simulink model "BikeManualControl"  (R2023b)
settings: Solver=VariableStepAuto  StartTime=0.0  StopTime=20  RelTol=1e-3
InitFcn:
  | run("config.m")
  | run("tracks\track_loader.mlx")
values from neighbouring files (symbols this model uses):
  angleFF = (lambda)    [INIT_BlueBike.m]    (also in config.m)
  angleRF = angleRF * (180/pi)    [INIT_BlueBike.m]    (also in config.m)
  b_contact_RW = 2e3    (= 2000)    [INIT_BlueBike.m]    (also in config.m)
  C_F_alpha = 1e3    (= 1000)    [INIT_BlueBike.m]    (also in config.m)
  C_F_kappa = 1e3    (= 1000)    [INIT_BlueBike.m]    (also in config.m)
  CM_phi = 0.3    [INIT_BlueBike.m]    (also in config.m)
  Dtheta0 = v0 / radiusRW    (= 0)    [INIT_BlueBike.m]    (also in config.m)
  Dtheta0_FW = v0 / radiusFW    (= 0)    [INIT_BlueBike.m]    (also in config.m)
  epsilon = 1e-2    (= 0.01)    [INIT_BlueBike.m]    (also in config.m)
  g = 9.81    [INIT_BlueBike.m]    (also in config.m)
  isoCameraAimX = (1/2)*w + 0.75    (= 1.267)    [INIT_BlueBike.m]    (also in config.m)
  isoCameraX = -2    [INIT_BlueBike.m]    (also in config.m)
  isoCameraY = -1.0    (= -1)    [INIT_BlueBike.m]    (also in config.m)
  isoCameraZ = -2*w    (= -2.068)    [INIT_BlueBike.m]    (also in config.m)
  k_contact_FW = 1e5    (= 100000)    [INIT_BlueBike.m]    (also in config.m)
  k_contact_RW = 1e5    (= 100000)    [INIT_BlueBike.m]    (also in config.m)
  lengthFF = frontHinge / (sind(lambda))    [INIT_BlueBike.m]    (also in config.m)
  lengthRF = sqrt((w-frontHinge)^2 + adj^2)    [INIT_BlueBike.m]    (also in config.m)
  lengthRW = 0.03    [INIT_BlueBike.m]    (also in config.m)
  massRW = 2    [INIT_BlueBike.m]    (also in config.m)
  max_rw_t = 10.0    (= 10)    [INIT_BlueBike.m]    (also in config.m = 20)
  max_steer_t = 5.0    (= 5)    [INIT_BlueBike.m]    (also in config.m)
  mB = 15    [INIT_BlueBike.m]    (also in config.m)
  mH = 5    [INIT_BlueBike.m]    (also in config.m)
  radiusFW = 0.325    [INIT_BlueBike.m]    (also in config.m)
  radiusRW = 0.32    [INIT_BlueBike.m]    (also in config.m)
  sigma = 0.12    [INIT_BlueBike.m]    (also in config.m)
  topViewX = -4.5*w    (= -4.653)    [INIT_BlueBike.m]    (also in config.m)
  topViewY = 0*w    (= 0)    [INIT_BlueBike.m]    (also in config.m)
  topViewZ = 1*w    (= 1.034)    [INIT_BlueBike.m]    (also in config.m)
  xPla = 3e3    (= 3000)    [INIT_BlueBike.m]    (also in config.m)
  yPla = 3e3    (= 3000)    [INIT_BlueBike.m]    (also in config.m)
  zPla = 0.01    [INIT_BlueBike.m]    (also in config.m)
undefined symbols (not defined in the file or in its folder): Cylinder, Parts_Lib, X, Y, Z
libraries: sm_lib x78, nesl_utility x32, vrlib x14, simulink x3
(part 4 of 4)

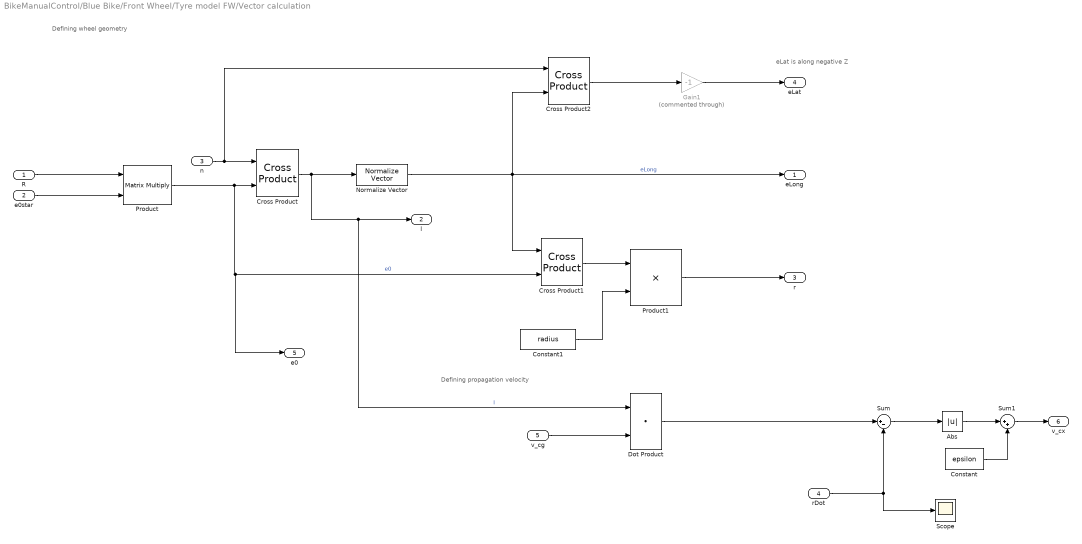
== system BikeManualControl/Blue Bike/Front Wheel/Tyre model FW/Vector calculation ==
  note: eLat is along
      | negative Z
  note: Defining wheel geometry
  note: Defining propagation velocity
  R : Inport
  e0star : Inport  Port=2
  n : Inport  Port=3
  rDot : Inport  Port=4
  v_cg : Inport  Port=5
  Abs : Abs  ZeroCross=off  SaturateOnIntegerOverflow=off
  Constant : Constant  Value=epsilon
  Constant1 : Constant  Value=radius
  Cross Product : vrlib/Utilities/Cross Product
  Cross Product1 : vrlib/Utilities/Cross Product
  Cross Product2 : vrlib/Utilities/Cross Product
  Dot Product : DotProduct  OutDataTypeStr=Inherit: Inherit via internal rule
  Gain1 : Gain  Commented=through  Gain=-1
  Normalize Vector : vrlib/Utilities/Normalize Vector  maxzero=0
  Product : Product  Multiplication=Matrix(*)
  Product1 : Product
  Scope : Scope
  Sum : Sum  Inputs=|+-
  Sum1 : Sum  Inputs=|++
  eLong : Outport  VectorParamsAs1DForOutWhenUnconnected=off
  l : Outport  Port=2  VectorParamsAs1DForOutWhenUnconnected=off
  r : Outport  Port=3  VectorParamsAs1DForOutWhenUnconnected=off
  eLat : Outport  Port=4  VectorParamsAs1DForOutWhenUnconnected=off
  e0 : Outport  Port=5  VectorParamsAs1DForOutWhenUnconnected=off
  v_cx : Outport  Port=6  VectorParamsAs1DForOutWhenUnconnected=off
  wires:
  rDot/1 -> Scope/1, Sum/2
  Constant1/1 -> Product1/2
  Gain1/1 -> eLat/1
  Product1/1 -> r/1
  Constant/1 -> Sum1/2
  Sum1/1 -> v_cx/1
  Abs/1 -> Sum1/1
  Sum/1 -> Abs/1
  Dot Product/1 -> Sum/1
  v_cg/1 -> Dot Product/2
  Cross Product2/1 -> Gain1/1
  Cross Product1/1 -> Product1/1
  Normalize Vector/1 -> Cross Product1/1, Cross Product2/2, eLong/1  "eLong"
  Cross Product/1 -> Normalize Vector/1, l/1, Dot Product/1  "l"
  n/1 -> Cross Product/1, Cross Product2/1
  Product/1 -> Cross Product/2, e0/1, Cross Product1/2  "e0"
  e0star/1 -> Product/2
  R/1 -> Product/1

== system BikeManualControl/Blue Bike/Front Wheel/Tyre model FW/Verticle force ==
  x_cg : Inport
  v_s : Inport  Port=2
  r : Inport  Port=3
  n : Inport  Port=4
  Dot Product : DotProduct  OutDataTypeStr=Inherit: Inherit via internal rule
  Dot Product1 : DotProduct  OutDataTypeStr=Inherit: Inherit via internal rule
  Gain : Gain  Gain=-k_contact
  Gain1 : Gain  Gain=-b_contact
  Initial position of CP from ground : Constant  Value=[0 0 0]
  Product : Product
  Scope1 : Scope
  Sum : Sum  Inputs=|++
  Sum1 : Sum  Inputs=|+-
  Sum2 : Sum
  Fn : Outport  VectorParamsAs1DForOutWhenUnconnected=off
  FnDisk : Outport  Port=2  VectorParamsAs1DForOutWhenUnconnected=off
  wires:
  Sum2/1 -> Product/1, Scope1/1, Fn/1
  Product/1 -> FnDisk/1
  Gain1/1 -> Sum2/2
  Dot Product/1 -> Gain/1  "pen"
  Gain/1 -> Sum2/1
  r/1 -> Sum/2
  n/1 -> Dot Product/2, Dot Product1/1, Product/2
  Dot Product1/1 -> Gain1/1  "pentration velocity"
  v_s/1 -> Dot Product1/2
  Sum1/1 -> Dot Product/1
  Initial position of CP from ground/1 -> Sum1/2
  Sum/1 -> Sum1/1  "CP position from ground"
  x_cg/1 -> Sum/1

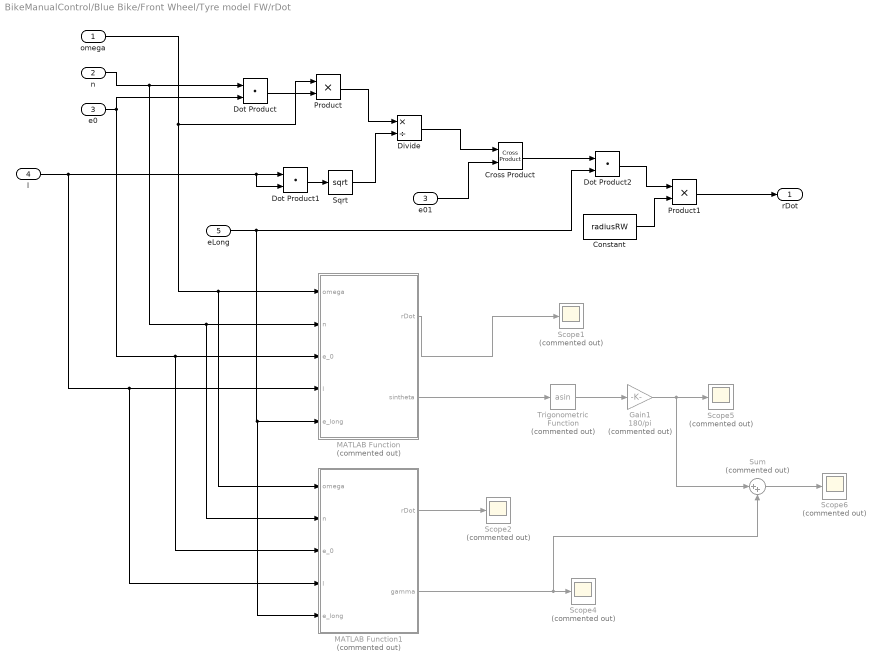
== system BikeManualControl/Blue Bike/Front Wheel/Tyre model FW/rDot ==
  omega : Inport
  n : Inport  Port=2
  e0 : Inport  Port=3
  l : Inport  Port=4
  eLong : Inport  Port=5
  Constant : Constant  Value=radiusRW
  Cross Product : vrlib/Utilities/Cross Product
  Divide : Product  Inputs=*/
  Dot Product : DotProduct  OutDataTypeStr=Inherit: Inherit via internal rule
  Dot Product1 : DotProduct  OutDataTypeStr=Inherit: Inherit via internal rule
  Dot Product2 : DotProduct  OutDataTypeStr=Inherit: Inherit via internal rule
  Gain1 : Gain  Commented=on  Gain=180/pi
  MATLAB Function : MATLAB Function  Commented=on  TreatAsAtomicUnit=on
  MATLAB Function1 : MATLAB Function  Commented=on  TreatAsAtomicUnit=on
  Product : Product
  Product1 : Product
  Scope{1..2,4..6} (5 alike) : Scope  Commented=on
  Sqrt : Sqrt
  Sum : Sum  Commented=on  Inputs=|++
  Trigonometric Function : Trigonometry  Commented=on  Operator=asin
  e01 : InportShadow  Port=3
  rDot : Outport  VectorParamsAs1DForOutWhenUnconnected=off
  wires:
  Sum/1 -> Scope6/1
  Gain1/1 -> Scope5/1, Sum/1
  Trigonometric Function/1 -> Gain1/1
  MATLAB Function/2(sintheta) -> Trigonometric Function/1
  MATLAB Function1/2(gamma) -> Scope4/1, Sum/2
  Product1/1 -> rDot/1
  MATLAB Function1/1(rDot) -> Scope2/1
  MATLAB Function/1(rDot) -> Scope1/1
  Constant/1 -> Product1/2
  Dot Product2/1 -> Product1/1
  eLong/1 -> Dot Product2/2, MATLAB Function/5(e_long), MATLAB Function1/5(e_long)
  Cross Product/1 -> Dot Product2/1
  e01/1 -> Cross Product/2
  Divide/1 -> Cross Product/1
  Sqrt/1 -> Divide/2
  Dot Product1/1 -> Sqrt/1
  l/1 -> Dot Product1/1, Dot Product1/2, MATLAB Function/4(l), MATLAB Function1/4(l)
  Product/1 -> Divide/1
  omega/1 -> Product/1, MATLAB Function/1(omega), MATLAB Function1/1(omega)
  Dot Product/1 -> Product/2
  e0/1 -> Dot Product/2, MATLAB Function/3(e_0), MATLAB Function1/3(e_0)
  n/1 -> Dot Product/1, MATLAB Function/2(n), MATLAB Function1/2(n)

== system BikeManualControl/Blue Bike/Rear Wheel/Tyre model/Camber thrust ==
  Fn : Inport
  eLat : Inport  Port=2
  n : Inport  Port=3
  e0 : Inport  Port=4
  Abs : Abs  ZeroCross=off  SaturateOnIntegerOverflow=off
  Compare To Constant : simulink/Logic and Bit Operations/Compare To Constant  relop=>=  const=0.9848  OutDataTypeStr=boolean
  Derivative : Derivative
  Dot Product1 : DotProduct  OutDataTypeStr=Inherit: Inherit via internal rule
  Product : Product
  Product1 : Product
  Scope1 : Scope
  Stop Simulation : Stop
  camber : Outport  VectorParamsAs1DForOutWhenUnconnected=off
  tag scope: Dphi=global, Lean=global
  wires:
  Fn/1 -> Product/1
  Product/1 -> Product1/1
  eLat/1 -> Product1/2
  Product1/1 -> Scope1/1, camber/1
  n/1 -> Dot Product1/1
  e0/1 -> Dot Product1/2
  Dot Product1/1 -> Derivative/1, [Lean], Abs/1, Product/2  "sin_gamma"
  Compare To Constant/1 -> Stop Simulation/1
  Abs/1 -> Compare To Constant/1
  Derivative/1 -> [Dphi]

== system BikeManualControl/Blue Bike/Rear Wheel/Tyre model/Force and moments block ==
  F_long : Inport
  F_lat : Inport  Port=2
  FnDisk : Inport  Port=3
  r : Inport  Port=4
  R : Inport  Port=5
  camber : Inport  Port=6
  phi_t : Inport  Port=7
  Add : Sum  Inputs=4
  Add1 : Sum
  Cross Product : vrlib/Utilities/Cross Product
  Demux : Demux  Outputs=3
  Demux1 : Demux  Outputs=3
  Product : Product  Inputs=/*  Multiplication=Matrix(*)
  Product1 : Product  Inputs=/*  Multiplication=Matrix(*)
  Scope : Scope  NumInputPorts=3
  Scope1 : Scope  NumInputPorts=3
  F : Outport  VectorParamsAs1DForOutWhenUnconnected=off
  M : Outport  Port=2  VectorParamsAs1DForOutWhenUnconnected=off
  wires:
  Add/1 -> Cross Product/2, Product/2
  R/1 -> Product1/1, Product/1
  Demux/3 -> Scope/3  "Mz"
  Demux/2 -> Scope/2  "My"
  Demux/1 -> Scope/1  "Mx"
  Cross Product/1 -> Add1/1
  camber/1 -> Add/4
  Product/1 -> Demux1/1, F/1
  Demux1/3 -> Scope1/3  "Fz"
  Demux1/2 -> Scope1/2  "Fy"
  Demux1/1 -> Scope1/1  "Fx"
  F_long/1 -> Add/2
  F_lat/1 -> Add/3
  Add1/1 -> Product1/2
  Product1/1 -> M/1, Demux/1
  r/1 -> Cross Product/1
  phi_t/1 -> Add1/2
  FnDisk/1 -> Add/1

== system BikeManualControl/Blue Bike/Rear Wheel/Tyre model/Lateral slip with relaxation ==
  v_s : Inport
  eLat : Inport  Port=2
  v_cx : Inport  Port=3
  eLong : Inport  Port=4
  Dot Product : DotProduct  OutDataTypeStr=Inherit: Inherit via internal rule
  Gain : Gain  Gain=1/sigma
  Gain1 : Gain  Gain=-C_F_alpha
  Integrator : Integrator
  Product : Product
  Product1 : Product
  Sum : Sum  Inputs=|+-
  F_Lat : Outport  VectorParamsAs1DForOutWhenUnconnected=off
  wires:
  v_s/1 -> Dot Product/1
  eLat/1 -> Product1/2, Dot Product/2
  Product/1 -> Sum/2
  Sum/1 -> Gain/1
  Gain/1 -> Integrator/1
  Integrator/1 -> Gain1/1, Product/2  "alpha_F"
  Gain1/1 -> Product1/1
  Product1/1 -> F_Lat/1
  v_cx/1 -> Product/1
  Dot Product/1 -> Sum/1  "s2"

== system BikeManualControl/Blue Bike/Rear Wheel/Tyre model/Longitudinal slip with relaxation ==
  v_s : Inport
  eLong : Inport  Port=2
  v_cx : Inport  Port=3
  Dot Product : DotProduct  OutDataTypeStr=Inherit: Inherit via internal rule
  Gain : Gain  Gain=1/sigma
  Gain1 : Gain  Gain=-C_F_kappa
  Integrator : Integrator
  Product : Product
  Product1 : Product
  Scope : Scope
  Scope1 : Scope
  Scope2 : Scope
  Sum : Sum  Inputs=|+-
  F_Long : Outport  VectorParamsAs1DForOutWhenUnconnected=off
  wires:
  v_s/1 -> Dot Product/1
  eLong/1 -> Product1/2, Dot Product/2
  Dot Product/1 -> Scope/1, Sum/1  "s1"
  Product/1 -> Sum/2
  Sum/1 -> Gain/1
  Gain/1 -> Integrator/1
  Integrator/1 -> Scope1/1, Gain1/1, Product/2  "kappa_F"
  Gain1/1 -> Product1/1
  Product1/1 -> Scope2/1, F_Long/1
  v_cx/1 -> Product/1

== system BikeManualControl/Blue Bike/Rear Wheel/Tyre model/Sensing ==
  PS-Simulink Converter{,1..9} (10 alike) : nesl_utility/PS-Simulink Converter  PhysicalDomain=network_engine_domain  SubClassName=ps_output  LeftPortType=input  RightPortType=output  PseudoPeriodic=off  Frequencies=[]  VectorFormat=1-D array  Unit=1  AffineConversion=off
  Transform Sensor : sm_lib/Frames and Transforms/Transform Sensor  MeasurementFrame=World  RotationSequence=XYX  SenseAngle=off  SenseAxis=off  SenseQ=off  SenseR=on  SenseRotationSequence=off  SenseOmegaX=on  SenseOmegaY=on  SenseOmegaZ=on  SenseOmega=off  SenseQDot=off  SenseRDot=off  SenseRotationSequenceDot=off  SenseAlphaX=off  SenseAlphaY=off  SenseAlphaZ=off  SenseAlpha=off  SenseQDDot=off  SenseRDDot=off  SenseX=on  SenseY=on  SenseZ=on  SenseXYZ=off  SenseRad=off  SenseAzim=off  SenseDist=off  SenseInc=off  SenseXDot=on  SenseYDot=on  SenseZDot=on  SenseXYZDot=off  SenseRadDot=off  SenseAzimDot=off  SenseDistDot=off  SenseIncDot=off  SenseXDDot=off  SenseYDDot=off  SenseZDDot=off  SenseXYZDDot=off  SenseRadDDot=off  SenseAzimDDot=off  SenseDistDDot=off  SenseIncDDot=off
  Wheel : PMIOPort  Side=Left
  Plane : PMIOPort  Port=2  Side=Left
  R : Outport  VectorParamsAs1DForOutWhenUnconnected=off
  x : Outport  Port=2  VectorParamsAs1DForOutWhenUnconnected=off
  y : Outport  Port=3  VectorParamsAs1DForOutWhenUnconnected=off
  z : Outport  Port=4  VectorParamsAs1DForOutWhenUnconnected=off
  vx : Outport  Port=5  VectorParamsAs1DForOutWhenUnconnected=off
  vy : Outport  Port=6  VectorParamsAs1DForOutWhenUnconnected=off
  vz : Outport  Port=7  VectorParamsAs1DForOutWhenUnconnected=off
  wx : Outport  Port=8  VectorParamsAs1DForOutWhenUnconnected=off
  wy : Outport  Port=9  VectorParamsAs1DForOutWhenUnconnected=off
  wz : Outport  Port=10  VectorParamsAs1DForOutWhenUnconnected=off
  wires:
  PS-Simulink Converter2/1 -> wy/1
  PS-Simulink Converter8/1 -> vy/1
  PS-Simulink Converter9/1 -> vz/1
  PS-Simulink Converter1/1 -> wx/1
  PS-Simulink Converter4/1 -> x/1
  PS-Simulink Converter7/1 -> vx/1
  PS-Simulink Converter3/1 -> wz/1
  PS-Simulink Converter5/1 -> y/1
  PS-Simulink Converter6/1 -> z/1
  PS-Simulink Converter/1 -> R/1
  connections:
  PS-Simulink Converter1/LConn1 -- Transform Sensor/RConn3
  PS-Simulink Converter4/LConn1 -- Transform Sensor/RConn6
  PS-Simulink Converter3/LConn1 -- Transform Sensor/RConn5
  PS-Simulink Converter9/LConn1 -- Transform Sensor/RConn11
  PS-Simulink Converter2/LConn1 -- Transform Sensor/RConn4
  PS-Simulink Converter6/LConn1 -- Transform Sensor/RConn8
  PS-Simulink Converter/LConn1 -- Transform Sensor/RConn2
  Transform Sensor/LConn1 -- Plane/RConn1
  Transform Sensor/RConn1 -- Wheel/RConn1
  PS-Simulink Converter5/LConn1 -- Transform Sensor/RConn7
  PS-Simulink Converter7/LConn1 -- Transform Sensor/RConn9
  PS-Simulink Converter8/LConn1 -- Transform Sensor/RConn10

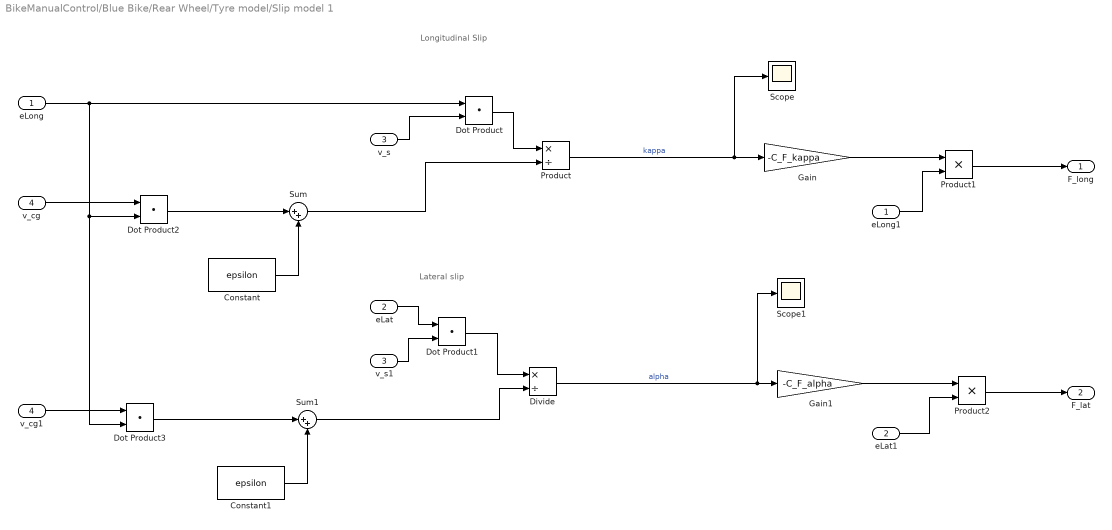
== system BikeManualControl/Blue Bike/Rear Wheel/Tyre model/Slip model 1 ==
  note: Lateral slip
  note: Longitudinal Slip
  eLong : Inport
  eLat : Inport  Port=2
  v_s : Inport  Port=3
  v_cg : Inport  Port=4
  Constant : Constant  Value=epsilon
  Constant1 : Constant  Value=epsilon
  Divide : Product  Inputs=*/
  Dot Product{,1..3} (4 alike) : DotProduct  OutDataTypeStr=Inherit: Inherit via internal rule
  Gain : Gain  Gain=-C_F_kappa
  Gain1 : Gain  Gain=-C_F_alpha
  Product : Product  Inputs=*/
  Product1 : Product
  Product2 : Product
  Scope : Scope
  Scope1 : Scope
  Sum : Sum  Inputs=|++
  Sum1 : Sum  Inputs=|++
  eLat1 : InportShadow  Port=2
  eLong1 : InportShadow
  v_cg1 : InportShadow  Port=4
  v_s1 : InportShadow  Port=3
  F_long : Outport  VectorParamsAs1DForOutWhenUnconnected=off
  F_lat : Outport  Port=2  VectorParamsAs1DForOutWhenUnconnected=off
  wires:
  eLong/1 -> Dot Product3/2, Dot Product2/2, Dot Product/1
  v_s/1 -> Dot Product/2
  Dot Product/1 -> Product/1
  Product/1 -> Scope/1, Gain/1  "kappa"
  eLat/1 -> Dot Product1/1
  v_s1/1 -> Dot Product1/2
  Dot Product1/1 -> Divide/1
  Divide/1 -> Scope1/1, Gain1/1  "alpha"
  Gain/1 -> Product1/1
  eLong1/1 -> Product1/2
  Gain1/1 -> Product2/1
  eLat1/1 -> Product2/2
  Product1/1 -> F_long/1
  Product2/1 -> F_lat/1
  Constant/1 -> Sum/2
  Sum/1 -> Product/2
  Constant1/1 -> Sum1/2
  Sum1/1 -> Divide/2
  v_cg/1 -> Dot Product2/1
  Dot Product2/1 -> Sum/1
  v_cg1/1 -> Dot Product3/1
  Dot Product3/1 -> Sum1/1

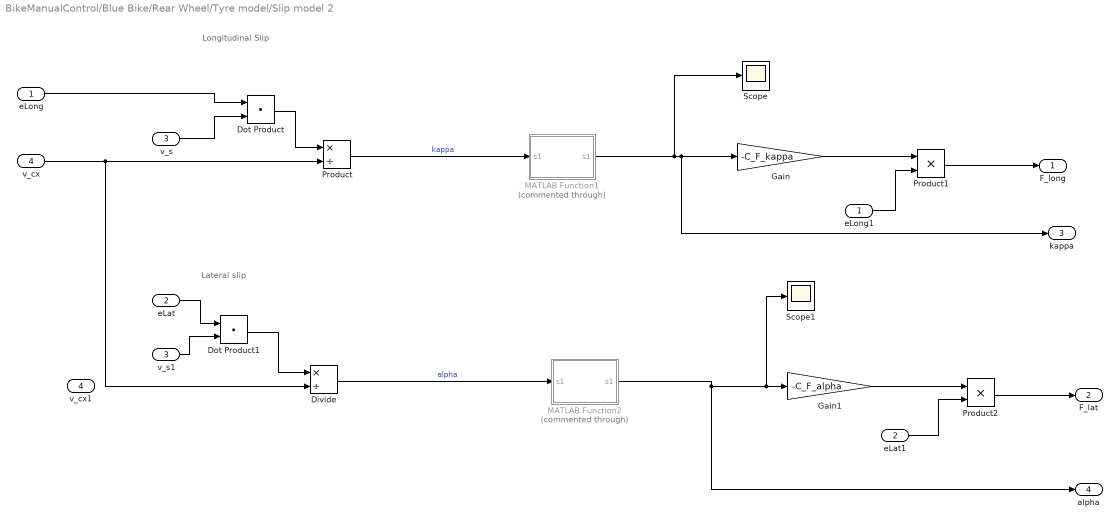
== system BikeManualControl/Blue Bike/Rear Wheel/Tyre model/Slip model 2 ==
  note: Lateral slip
  note: Longitudinal Slip
  eLong : Inport
  eLat : Inport  Port=2
  v_s : Inport  Port=3
  v_cx : Inport  Port=4
  Divide : Product  Inputs=*/
  Dot Product : DotProduct  OutDataTypeStr=Inherit: Inherit via internal rule
  Dot Product1 : DotProduct  OutDataTypeStr=Inherit: Inherit via internal rule
  Gain : Gain  Gain=-C_F_kappa
  Gain1 : Gain  Gain=-C_F_alpha
  MATLAB Function1 : MATLAB Function  Commented=through  TreatAsAtomicUnit=on
  MATLAB Function2 : MATLAB Function  Commented=through  TreatAsAtomicUnit=on
  Product : Product  Inputs=*/
  Product1 : Product
  Product2 : Product
  Scope : Scope
  Scope1 : Scope
  eLat1 : InportShadow  Port=2
  eLong1 : InportShadow
  v_cx1 : InportShadow  Port=4
  v_s1 : InportShadow  Port=3
  F_long : Outport  VectorParamsAs1DForOutWhenUnconnected=off
  F_lat : Outport  Port=2  VectorParamsAs1DForOutWhenUnconnected=off
  kappa : Outport  Port=3  VectorParamsAs1DForOutWhenUnconnected=off
  alpha : Outport  Port=4  VectorParamsAs1DForOutWhenUnconnected=off
  wires:
  eLong/1 -> Dot Product/1
  Dot Product/1 -> Product/1
  eLat/1 -> Dot Product1/1
  Dot Product1/1 -> Divide/1
  Divide/1 -> MATLAB Function2/1("s1 ")  "alpha"
  Gain/1 -> Product1/1
  eLong1/1 -> Product1/2
  Gain1/1 -> Product2/1
  eLat1/1 -> Product2/2
  Product1/1 -> F_long/1
  Product2/1 -> F_lat/1
  v_s/1 -> Dot Product/2
  v_s1/1 -> Dot Product1/2
  Product/1 -> MATLAB Function1/1("s1 ")  "kappa"
  v_cx/1 -> Divide/2, Product/2
  MATLAB Function1/1(s1) -> Scope/1, kappa/1, Gain/1
  MATLAB Function2/1(s1) -> alpha/1, Scope1/1, Gain1/1

== system BikeManualControl/Blue Bike/Rear Wheel/Tyre model/Slip velocity ==
  omega : Inport
  v_cg : Inport  Port=2
  r : Inport  Port=3
  Add : Sum
  Cross Product : vrlib/Utilities/Cross Product
  Scope : Scope
  v_s : Outport  VectorParamsAs1DForOutWhenUnconnected=off
  wires:
  omega/1 -> Cross Product/1
  Cross Product/1 -> Scope/1, Add/2  "v_r"
  r/1 -> Cross Product/2
  v_cg/1 -> Add/1  "V_x"
  Add/1 -> v_s/1

== system BikeManualControl/Blue Bike/Rear Wheel/Tyre model/Turn Slip ==
  omega : Inport
  n : Inport  Port=2
  v_cx : Inport  Port=3
  Dot Product : DotProduct  OutDataTypeStr=Inherit: Inherit via internal rule
  Gain : Gain  Gain=1/sigma
  Gain1 : Gain  Gain=-CM_phi
  Gain2 : Gain  Gain=-1
  Integrator : Integrator
  Product : Product
  Product1 : Product
  Product2 : Product  Inputs=*/
  Scope : Scope
  Scope1 : Scope
  Sum : Sum  Inputs=|+-
  phi_t : Outport  VectorParamsAs1DForOutWhenUnconnected=off
  wires:
  omega/1 -> Dot Product/1
  n/1 -> Product/2, Dot Product/2
  Dot Product/1 -> Gain2/1, Sum/1
  Sum/1 -> Gain/1
  Gain/1 -> Integrator/1
  Integrator/1 -> Product1/2, Gain1/1
  Gain1/1 -> Scope/1, Product/1
  Product/1 -> phi_t/1
  v_cx/1 -> Product2/2, Product1/1
  Product1/1 -> Sum/2
  Product2/1 -> Scope1/1
  Gain2/1 -> Product2/1

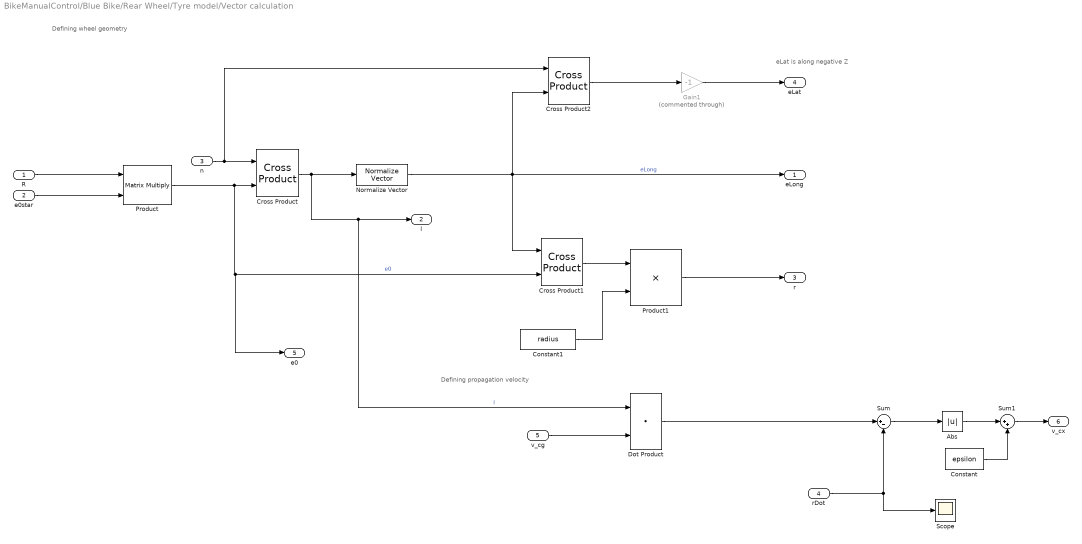
== system BikeManualControl/Blue Bike/Rear Wheel/Tyre model/Vector calculation ==
  note: Defining propagation velocity
  note: Defining wheel geometry
  note: eLat is along
      | negative Z
  R : Inport
  e0star : Inport  Port=2
  n : Inport  Port=3
  rDot : Inport  Port=4
  v_cg : Inport  Port=5
  Abs : Abs  ZeroCross=off  SaturateOnIntegerOverflow=off
  Constant : Constant  Value=epsilon
  Constant1 : Constant  Value=radius
  Cross Product : vrlib/Utilities/Cross Product
  Cross Product1 : vrlib/Utilities/Cross Product
  Cross Product2 : vrlib/Utilities/Cross Product
  Dot Product : DotProduct  OutDataTypeStr=Inherit: Inherit via internal rule
  Gain1 : Gain  Commented=through  Gain=-1
  Normalize Vector : vrlib/Utilities/Normalize Vector  maxzero=0
  Product : Product  Multiplication=Matrix(*)
  Product1 : Product
  Scope : Scope
  Sum : Sum  Inputs=|+-
  Sum1 : Sum  Inputs=|++
  eLong : Outport  VectorParamsAs1DForOutWhenUnconnected=off
  l : Outport  Port=2  VectorParamsAs1DForOutWhenUnconnected=off
  r : Outport  Port=3  VectorParamsAs1DForOutWhenUnconnected=off
  eLat : Outport  Port=4  VectorParamsAs1DForOutWhenUnconnected=off
  e0 : Outport  Port=5  VectorParamsAs1DForOutWhenUnconnected=off
  v_cx : Outport  Port=6  VectorParamsAs1DForOutWhenUnconnected=off
  wires:
  R/1 -> Product/1
  e0star/1 -> Product/2
  Product/1 -> Cross Product1/2, e0/1, Cross Product/2  "e0"
  n/1 -> Cross Product2/1, Cross Product/1
  Cross Product/1 -> Dot Product/1, l/1, Normalize Vector/1  "l"
  Normalize Vector/1 -> eLong/1, Cross Product2/2, Cross Product1/1  "eLong"
  Cross Product1/1 -> Product1/1
  Cross Product2/1 -> Gain1/1
  v_cg/1 -> Dot Product/2
  Dot Product/1 -> Sum/1
  Sum/1 -> Abs/1
  Abs/1 -> Sum1/1
  Sum1/1 -> v_cx/1
  Constant/1 -> Sum1/2
  Product1/1 -> r/1
  Gain1/1 -> eLat/1
  Constant1/1 -> Product1/2
  rDot/1 -> Sum/2, Scope/1

== system BikeManualControl/Blue Bike/Rear Wheel/Tyre model/Verticle force ==
  x_cg : Inport
  v_s : Inport  Port=2
  r : Inport  Port=3
  n : Inport  Port=4
  Dot Product : DotProduct  OutDataTypeStr=Inherit: Inherit via internal rule
  Dot Product1 : DotProduct  OutDataTypeStr=Inherit: Inherit via internal rule
  Gain : Gain  Gain=-k_contact
  Gain1 : Gain  Gain=-b_contact
  Initial position of CP from ground : Constant  Value=[0 0 0]'
  Product : Product
  Scope1 : Scope
  Sum : Sum  Inputs=|++
  Sum1 : Sum  Inputs=|+-
  Sum2 : Sum
  Fn : Outport  VectorParamsAs1DForOutWhenUnconnected=off
  FnDisk : Outport  Port=2  VectorParamsAs1DForOutWhenUnconnected=off
  wires:
  x_cg/1 -> Sum/1
  Sum/1 -> Sum1/1  "CP position from ground"
  Initial position of CP from ground/1 -> Sum1/2
  Sum1/1 -> Dot Product/1
  v_s/1 -> Dot Product1/2
  Dot Product1/1 -> Gain1/1  "pentration velocity"
  n/1 -> Product/2, Dot Product1/1, Dot Product/2
  r/1 -> Sum/2
  Gain/1 -> Sum2/1
  Dot Product/1 -> Gain/1  "pen"
  Gain1/1 -> Sum2/2
  Product/1 -> FnDisk/1
  Sum2/1 -> Fn/1, Product/1, Scope1/1

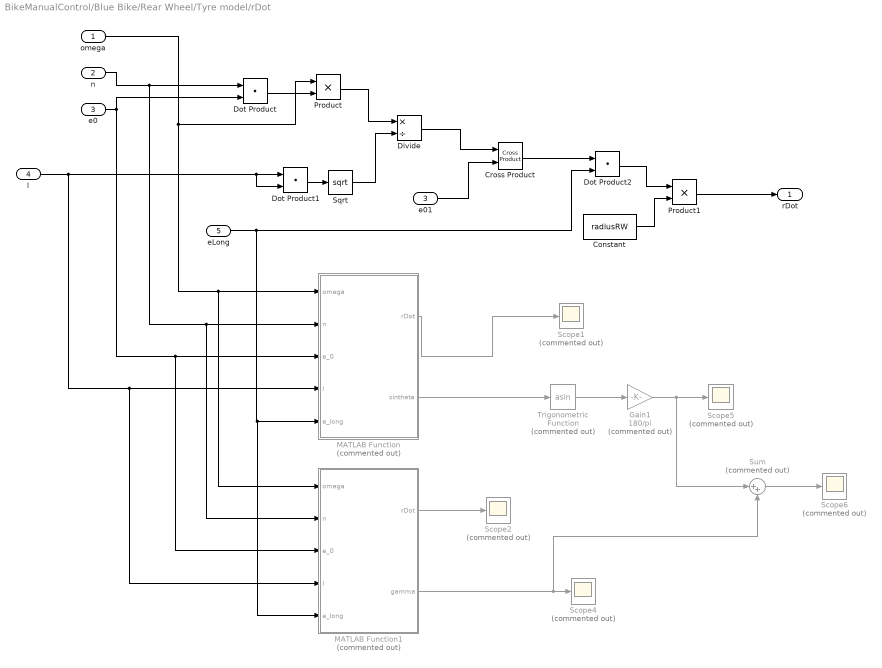
== system BikeManualControl/Blue Bike/Rear Wheel/Tyre model/rDot ==
  omega : Inport
  n : Inport  Port=2
  e0 : Inport  Port=3
  l : Inport  Port=4
  eLong : Inport  Port=5
  Constant : Constant  Value=radiusRW
  Cross Product : vrlib/Utilities/Cross Product
  Divide : Product  Inputs=*/
  Dot Product : DotProduct  OutDataTypeStr=Inherit: Inherit via internal rule
  Dot Product1 : DotProduct  OutDataTypeStr=Inherit: Inherit via internal rule
  Dot Product2 : DotProduct  OutDataTypeStr=Inherit: Inherit via internal rule
  Gain1 : Gain  Commented=on  Gain=180/pi
  MATLAB Function : MATLAB Function  Commented=on  TreatAsAtomicUnit=on
  MATLAB Function1 : MATLAB Function  Commented=on  TreatAsAtomicUnit=on
  Product : Product
  Product1 : Product
  Scope{1..2,4..6} (5 alike) : Scope  Commented=on
  Sqrt : Sqrt
  Sum : Sum  Commented=on  Inputs=|++
  Trigonometric Function : Trigonometry  Commented=on  Operator=asin
  e01 : InportShadow  Port=3
  rDot : Outport  VectorParamsAs1DForOutWhenUnconnected=off
  wires:
  n/1 -> MATLAB Function1/2(n), MATLAB Function/2(n), Dot Product/1
  e0/1 -> MATLAB Function1/3(e_0), MATLAB Function/3(e_0), Dot Product/2
  Dot Product/1 -> Product/2
  omega/1 -> MATLAB Function1/1(omega), MATLAB Function/1(omega), Product/1
  Product/1 -> Divide/1
  l/1 -> MATLAB Function1/4(l), MATLAB Function/4(l), Dot Product1/2, Dot Product1/1
  Dot Product1/1 -> Sqrt/1
  Sqrt/1 -> Divide/2
  Divide/1 -> Cross Product/1
  e01/1 -> Cross Product/2
  Cross Product/1 -> Dot Product2/1
  eLong/1 -> MATLAB Function1/5(e_long), MATLAB Function/5(e_long), Dot Product2/2
  Dot Product2/1 -> Product1/1
  Constant/1 -> Product1/2
  MATLAB Function/1(rDot) -> Scope1/1
  MATLAB Function1/1(rDot) -> Scope2/1
  Product1/1 -> rDot/1
  MATLAB Function1/2(gamma) -> Sum/2, Scope4/1
  MATLAB Function/2(sintheta) -> Trigonometric Function/1
  Trigonometric Function/1 -> Gain1/1
  Gain1/1 -> Sum/1, Scope5/1
  Sum/1 -> Scope6/1

== matlab function BikeManualControl/Blue Bike/Rear Wheel/Tyre model/rDot/MATLAB Function1 ==
  data: rDot output; omega input; n input; e_0 input; l input; e_long input; gamma output
function [rDot,gamma] = fcn(omega,n,e_0,l,e_long)

sinGamma = dot(n,e_0);
firstTerm = (omega*sinGamma)/norm(l);
crossProd = cross(firstTerm,e_0);
rDot = dot(crossProd,e_long);
gamma = asind(sinGamma);

== matlab function BikeManualControl/Blue Bike/Rear Wheel/Tyre model/rDot/MATLAB Function ==
  data: rDot output; omega input; n input; e_0 input; l input; e_long input; radiusRW parameter; sintheta output
function [rDot,sintheta]  = fcn(omega,n,e_0,l,e_long, radiusRW)

sintheta = norm(l);
dotProd = dot(n,e_0);
firstTerm = omega * dotProd / sintheta;
crossProd = cross(firstTerm,e_0);
dotProd2 = dot(crossProd,e_long);
rDot = radiusRW * dotProd2;
% thetad = asind(sintheta) * (180/pi);

== matlab function BikeManualControl/Blue Bike/Rear Wheel/Tyre model/Slip model 2/MATLAB Function1 ==
  data: s1 input; s1 output
function s1 = fcn(s1)

if s1 < 1e-7 && s1 > -1e-7
    s1 = 0;
else
    s1 = s1;
end

== matlab function BikeManualControl/Blue Bike/Rear Wheel/Tyre model/Slip model 2/MATLAB Function2 ==
  data: s1 input; s1 output
function s1 = fcn(s1)

if s1 < 1e-8 && s1 > -1e-8
    s1 = 0;
else
    s1 = s1;
end

== matlab function BikeManualControl/Blue Bike/Front Wheel/Tyre model FW/Slip model 2/MATLAB Function1 ==
  data: s1 input; s1 output
function s1 = fcn(s1)

if s1 < 1e-7 && s1 > -1e-7
    s1 = 0;
else
    s1 = s1;
end

== matlab function BikeManualControl/Blue Bike/Front Wheel/Tyre model FW/Slip model 2/MATLAB Function2 ==
  data: s1 input; s1 output
function s1 = fcn(s1)

if s1 < 1e-8 && s1 > -1e-8
    s1 = 0;
else
    s1 = s1;
end

== matlab function BikeManualControl/Blue Bike/Front Wheel/Tyre model FW/rDot/MATLAB Function ==
  data: rDot output; omega input; n input; e_0 input; l input; e_long input; radiusRW parameter; sintheta output
function [rDot,sintheta]  = fcn(omega,n,e_0,l,e_long, radiusRW)

sintheta = norm(l);
dotProd = dot(n,e_0);
firstTerm = omega * dotProd / sintheta;
crossProd = cross(firstTerm,e_0);
dotProd2 = dot(crossProd,e_long);
rDot = radiusRW * dotProd2;
% thetad = asind(sintheta) * (180/pi);

== matlab function BikeManualControl/Blue Bike/Front Wheel/Tyre model FW/rDot/MATLAB Function1 ==
  data: rDot output; omega input; n input; e_0 input; l input; e_long input; gamma output
function [rDot,gamma] = fcn(omega,n,e_0,l,e_long)

sinGamma = dot(n,e_0);
firstTerm = (omega*sinGamma)/norm(l);
crossProd = cross(firstTerm,e_0);
rDot = dot(crossProd,e_long);
gamma = asind(sinGamma);
